simulink model "pendolo_modelfunction"  (R2020b)
settings: Solver=VariableStepAuto  StartTime=0.0  StopTime=20  RelTol=1e-3
settings Model: Creator=Lenovo  LastModifiedBy=Lenovo

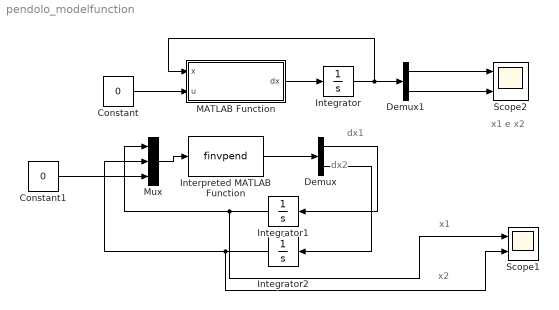
== system pendolo_modelfunction ==
  note: x1
  note: x2
  note: dx2
  note: dx1
  note: x1 e x2
  Constant : Constant  Value=0
  Constant1 : Constant  Value=0
  Demux : Demux  Outputs=2
  Demux1 : Demux  Outputs=2
  Integrator : Integrator  InitialCondition=[0.7;0]
  Integrator1 : Integrator  InitialCondition=0.7
  Integrator2 : Integrator
  Interpreted MATLAB Function : MATLABFcn  MATLABFcn=finvpend
  MATLAB Function : MATLAB Function  TreatAsAtomicUnit=on
  Mux : Mux  Inputs=3
  Scope1 : Scope  NumInputPorts=2
  Scope2 : Scope  NumInputPorts=2
  wires:
  Constant/1 -> MATLAB Function/2(u)
  MATLAB Function/1(dx) -> Integrator/1
  Integrator/1 -> Demux1/1, MATLAB Function/1(x)
  Interpreted MATLAB Function/1 -> Demux/1
  Demux/1 -> Integrator1/1
  Mux/1 -> Interpreted MATLAB Function/1
  Integrator1/1 -> Scope1/1, Mux/1
  Integrator2/1 -> Scope1/2, Mux/2
  Constant1/1 -> Mux/3
  Demux/2 -> Integrator2/1
  Demux1/1 -> Scope2/1
  Demux1/2 -> Scope2/2

== matlab function pendolo_modelfunction/MATLAB Function ==
  data: x input; u input; dx output
function dx = pendolo_inverso(x,u)
%#codegen
a=0.25;
k=4.5;
m=1;
L=0.5;
g=9.81;

x1=x(1);
x2=x(2);


dx=[x2;-a/(m*L^2)*x2-k/(m*L^2)*x1+g/L*sin(x1)+u/(m*L^2)];
